simulink model "Oversamplingcircuit"  (R2014a)
settings: Solver=ode3  StartTime=0.0  StopTime=1/441*10  FixedStep=1/(44100*16)  RelTol=1e-3
libraries: dsparch4 x1
settings Model: Creator=Administratör  LastModifiedBy=Administratör

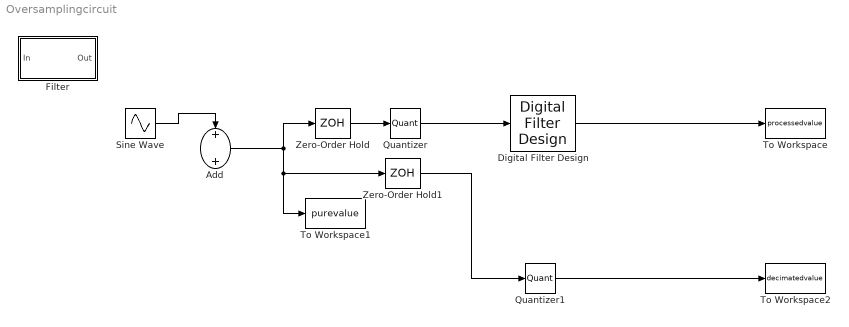
== system Oversamplingcircuit ==
  Add : Sum
  Digital Filter Design : dsparch4/Digital Filter Design  mwdsp_browser_bugfix_var=off
  Filter : Subsystem  Tag=BlockMethodSubSystem
  Quantizer : Quantizer  QuantizationInterval=2^-(2-1)  LinearizeAsGain=off
  Quantizer1 : Quantizer  QuantizationInterval=2^-(2-1)  LinearizeAsGain=off
  Sine Wave : Sin  Frequency=441*2*pi  SampleTime=0
  To Workspace : ToWorkspace  VariableName=processedvalue  SaveFormat=Structure With Time  SampleTime=-1
  To Workspace1 : ToWorkspace  VariableName=purevalue  SaveFormat=Structure With Time  SampleTime=-1
  To Workspace2 : ToWorkspace  VariableName=decimatedvalue  SaveFormat=Structure With Time  SampleTime=-1
  Zero-Order Hold : ZeroOrderHold  SampleTime=1/(44100*16)
  Zero-Order Hold1 : ZeroOrderHold  SampleTime=1/(44100)
  wires:
  Quantizer/1 -> Digital Filter Design/1
  Digital Filter Design/1 -> To Workspace/1
  Add/1 -> Zero-Order Hold1/1, To Workspace1/1, Zero-Order Hold/1
  Sine Wave/1 -> Add/1
  ? -> Add/2
  Zero-Order Hold/1 -> Quantizer/1
  Zero-Order Hold1/1 -> Quantizer1/1
  Quantizer1/1 -> To Workspace2/1

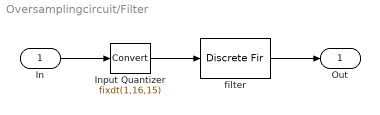
== system Oversamplingcircuit/Filter ==
  In : Inport
  Input Quantizer : DataTypeConversion  OutDataTypeStr=fixdt(1,16,15)  RndMeth=Round  SaturateOnIntegerOverflow=on
  filter : DiscreteFir  Coefficients=[-0.010731812447070192 -0.004089865405164087 -0.0042364647432413796 -0.0038429671792891114 -0.0027762818306671217 -0.00091969543572465503 0.0018154303662518635 0.0054667652665586677 0.010037181787807065 0.015458533769094673 0.021634483058161433 0.028373009418329393 0.035495643998727539 0.042710206325209582 0.049764523497556223 0.056369200980915121 0.062225046224720283 0.067083388405467043 0.070723681318964005 0.072989169604716742 0.073753517190912582 0.072989169604716742 0.070723681318964005 0.067083388405467043 0.062225046224720283 0.056369200980915121 0.049764523497556223 0.042710206325209582 0.035495643998727539 0.028373009418329393 0.021634483058161433 0.015458533769094673 0.010037181787807065 0.0054667652665586677 0.0018154303662518635 -0.00091969543572465503 -0.0027762818306671217 -0.0038429671792891114 -0.0042364647432413796 -0.004089865405164087 -0.010731812447070192]  InputProcessing=Columns as channels (frame based)  CoefDataTypeStr=fixdt(true,32,34)  ProductDataTypeStr=fixdt(true,47,49)  AccumDataTypeStr=fixdt(true,51,49)  OutDataTypeStr=fixdt(true,51,49)  RndMeth=Convergent
  Out : Outport
  wires:
  In/1 -> Input Quantizer/1
  Input Quantizer/1 -> filter/1
  filter/1 -> Out/1
